simulink model "ControlDigital_Observadores"  (R2016a)
settings: Solver=VariableStepAuto  StartTime=0.0  StopTime=50  RelTol=1e-3
values from neighbouring files (symbols this model uses):
  Ac_2 = [ALn-BLn*Kest-L*CLn+L*DLn*Kest, BLn*Ki - L*DLn*Ki ... (first row only)    [Control_MIMO_Observadores.m]    (also in Diseno_lqg_funcion_transferencia.m = Reg_2dof.a; Ejercicio_funcion_lqg.m = Reg_2dof.a)
  ALn = double(subs(AL,{a,b,c,d},{a1,b1,c1,d1}))    [Control_MIMO_Observadores.m]    (also in Control_MIMO_Observadores_Equilibrio.m)
  Bc_2 = [zeros(n,r),L ... (first row only)    [Control_MIMO_Observadores.m]    (also in Diseno_lqg_funcion_transferencia.m = Reg_2dof.b; Ejercicio_funcion_lqg.m = Reg_2dof.b)
  BLn = double(subs(BL,{a,b,c,d},{a1,b1,c1,d1}))    [Control_MIMO_Observadores.m]    (also in Control_MIMO_Observadores_Equilibrio.m)
  Cc_2 = [-Kest, Ki]    [Control_MIMO_Observadores.m]    (also in Diseno_lqg_funcion_transferencia.m = Reg_2dof.c; Ejercicio_funcion_lqg.m = Reg_2dof.c)
  CLn = [1 0 0 ... (first row only)    [Control_MIMO_Observadores.m]    (also in Control_MIMO_Observadores_Equilibrio.m)
  Dc_2 = zeros(p,2*r)    [Control_MIMO_Observadores.m]    (also in Diseno_lqg_funcion_transferencia.m = Reg_2dof.d; Ejercicio_funcion_lqg.m = Reg_2dof.d)
  DLn = [0 0 0 ... (first row only)    [Control_MIMO_Observadores.m]    (also in Control_MIMO_Observadores_Equilibrio.m)
  Kaw = [0 0 0 ... (first row only)    [Control_MIMO_Observadores.m]
  Kest = Kt(:,1:n)    [Control_MIMO_Observadores.m]
  Ki = -Kt(:,n+1:end)    [Control_MIMO_Observadores.m]
  L = (Grand*inv(X))'    [Control_MIMO_Observadores.m]    (also in Control_MIMO_Observadores_Equilibrio.m)
  sys_d2 = c2d(sys_c2,Tm)    [Control_MIMO_Observadores.m]
  Tm = 0.01    [Control_MIMO_Observadores.m]    (also in Control_MIMO_Observadores_Equilibrio.m)
  u10 = double((a1*x20 + b1*x10^2)/u20)    [Control_MIMO_Observadores.m]    (also in Control_MIMO_Observadores_Equilibrio.m)
  u20 = double(sqrt(c1*x30*x20))    [Control_MIMO_Observadores.m]    (also in Control_MIMO_Observadores_Equilibrio.m)
  u30 = double((d1*x30 - u10)/x10)    [Control_MIMO_Observadores.m]    (also in Control_MIMO_Observadores_Equilibrio.m)
  x10 = 2    [Control_MIMO_Observadores.m]    (also in Control_MIMO_Observadores_Equilibrio.m)
  x20 = 4    [Control_MIMO_Observadores.m]    (also in Control_MIMO_Observadores_Equilibrio.m)
  x30 = 4    [Control_MIMO_Observadores.m]    (also in Control_MIMO_Observadores_Equilibrio.m)
  xini = [0.5; -0.3; -0.7]    [Control_MIMO_Observadores_Equilibrio.m]
libraries: simulink x14, cstblocks x5
settings Model: Creator=Lenovo  LastModifiedBy=Lenovo

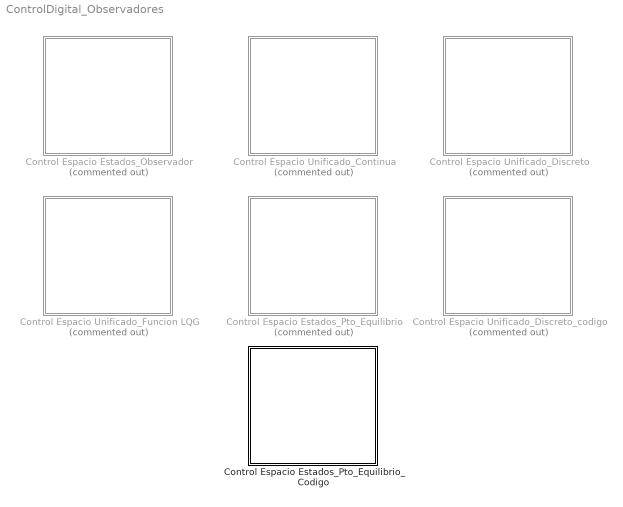
== system ControlDigital_Observadores ==
  Control Espacio Estados_Observador : Subsystem  Commented=on
  Control Espacio Estados_Pto_Equilibrio : Subsystem  Commented=on
  Control Espacio Estados_Pto_Equilibrio_Codigo : Subsystem
  Control Espacio Unificado_Continua : Subsystem  Commented=on
  Control Espacio Unificado_Discreto : Subsystem  Commented=on
  Control Espacio Unificado_Discreto_codigo : Subsystem  Commented=on
  Control Espacio Unificado_Funcion LQG : Subsystem  Commented=on

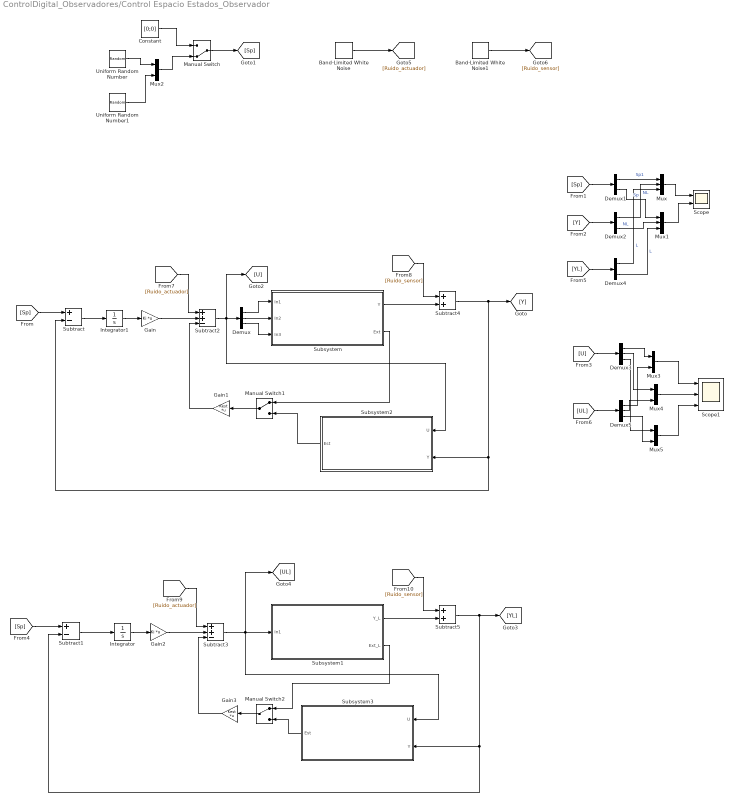
== system ControlDigital_Observadores/Control Espacio Estados_Observador ==
  Band-Limited White Noise : simulink/Sources/Band-Limited White Noise  Cov=[1e-6, 1e-7, 1e-6 ]  Ts=0.01  seed=[23341]
  Band-Limited White Noise1 : simulink/Sources/Band-Limited White Noise  Cov=[1e-6, 1e-6]  Ts=0.01  seed=[23341]
  Constant : Constant  Value=[0;0]
  Demux : Demux  Outputs=3
  Demux1 : Demux  Outputs=2
  Demux2 : Demux  Outputs=2
  Demux3 : Demux  Outputs=3
  Demux4 : Demux  Outputs=2
  Demux5 : Demux  Outputs=3
  Gain : Gain  Gain=Ki  Multiplication=Matrix(K*u)
  Gain1 : Gain  Gain=Kest  Multiplication=Matrix(K*u)
  Gain2 : Gain  Gain=Ki  Multiplication=Matrix(K*u)
  Gain3 : Gain  Gain=Kest  Multiplication=Matrix(K*u)
  Integrator : Integrator
  Integrator1 : Integrator
  Manual Switch : ManualSwitch  CurrentSetting=0
  Manual Switch1 : ManualSwitch
  Manual Switch2 : ManualSwitch
  Mux : Mux  Inputs=3
  Mux1 : Mux  Inputs=3
  Mux{2..5} (4 alike) : Mux  Inputs=2
  Scope : Scope  NumInputPorts=2
  Scope1 : Scope  NumInputPorts=3
  Subsystem : Subsystem
  Subsystem1 : Subsystem
  Subsystem2 : Subsystem
  Subsystem3 : Subsystem
  Subtract : Sum  Inputs=+-
  Subtract1 : Sum  Inputs=+-
  Subtract2 : Sum  Inputs=++-
  Subtract3 : Sum  Inputs=++-
  Subtract4 : Sum
  Subtract5 : Sum
  Uniform Random Number : UniformRandomNumber  Minimum=-0.3  Maximum=0.3  SampleTime=6
  Uniform Random Number1 : UniformRandomNumber  Minimum=-0.5  Maximum=0.5  SampleTime=13
  wires:
  Demux2/1 -> Mux/2  "NL"
  Demux2/2 -> Mux1/2  "NL"
  [Sp] -> Demux1/1
  [Sp] -> Subtract/1
  Demux/3 -> Subsystem/3(In3)
  Demux/2 -> Subsystem/2(In2)
  Constant/1 -> Manual Switch/1
  Manual Switch/1 -> [Sp]
  Demux1/1 -> Mux/1  "Sp1"
  Demux1/2 -> Mux1/1  "Sp"
  Demux/1 -> Subsystem/1(In1)
  [Y] -> Demux2/1
  Mux1/1 -> Scope/2
  Mux/1 -> Scope/1
  Mux5/1 -> Scope1/3
  Uniform Random Number/1 -> Mux2/1
  [Sp] -> Subtract1/1
  Demux5/1 -> Mux3/2
  [U] -> Demux3/1
  Demux5/3 -> Mux5/2
  [YL] -> Demux4/1
  Demux3/2 -> Mux4/1
  Demux3/1 -> Mux3/1
  Demux3/3 -> Mux5/1
  Demux5/2 -> Mux4/2
  Mux3/1 -> Scope1/1
  Mux4/1 -> Scope1/2
  Demux4/2 -> Mux1/3  "L"
  Uniform Random Number1/1 -> Mux2/2
  Demux4/1 -> Mux/3  "L"
  [UL] -> Demux5/1
  Mux2/1 -> Manual Switch/2
  Subtract2/1 -> Subsystem2/1(U), [U], Demux/1
  Manual Switch1/1 -> Gain1/1
  Subsystem/2(Ext) -> Manual Switch1/1
  Subsystem2/1(Est) -> Manual Switch1/2
  Subsystem3/1(Est) -> Manual Switch2/2
  Subsystem1/2(Ext_L) -> Manual Switch2/1
  Subtract1/1 -> Integrator/1
  Integrator1/1 -> Gain/1
  Subtract/1 -> Integrator1/1
  Band-Limited White Noise/1 -> [Ruido_actuador]
  Band-Limited White Noise1/1 -> [Ruido_sensor]
  Gain1/1 -> Subtract2/3
  Gain/1 -> Subtract2/2
  [Ruido_actuador] -> Subtract2/1
  Subtract4/1 -> [Y], Subsystem2/2(Y), Subtract/2
  Subsystem/1(Y) -> Subtract4/2
  [Ruido_sensor] -> Subtract4/1
  Subtract3/1 -> Subsystem3/1(U), [UL], Subsystem1/1(In1)
  Integrator/1 -> Gain2/1
  Gain3/1 -> Subtract3/3
  Gain2/1 -> Subtract3/2
  [Ruido_actuador] -> Subtract3/1
  Manual Switch2/1 -> Gain3/1
  Subsystem1/1(Y_L) -> Subtract5/2
  [Ruido_sensor] -> Subtract5/1
  Subtract5/1 -> Subsystem3/2(Y), Subtract1/2, [YL]

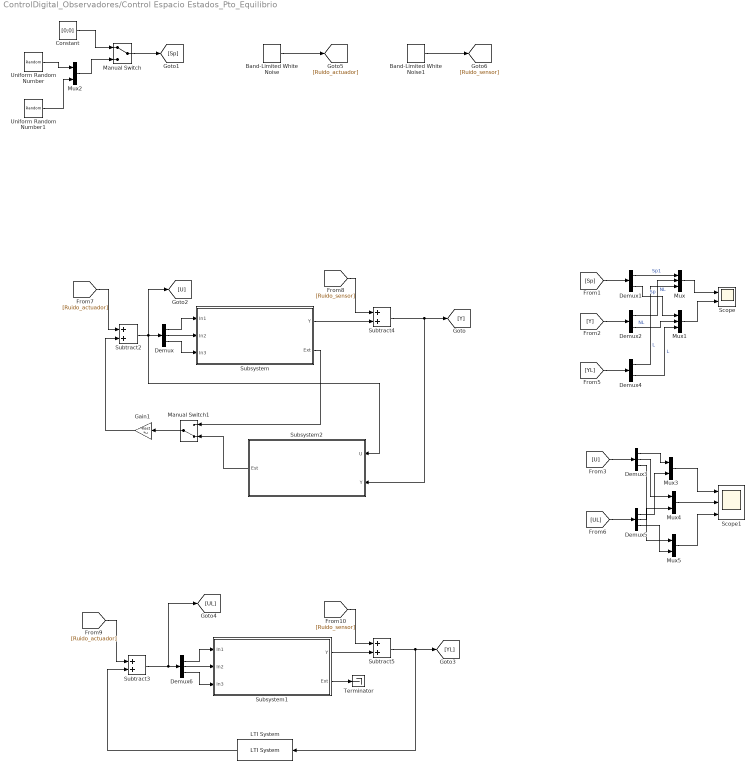
== system ControlDigital_Observadores/Control Espacio Estados_Pto_Equilibrio ==
  Band-Limited White Noise : simulink/Sources/Band-Limited White Noise  Cov=[1e-7, 1e-8, 1e-7 ]  Ts=1e-3  seed=[23341]
  Band-Limited White Noise1 : simulink/Sources/Band-Limited White Noise  Cov=[1e-7, 1e-7]  Ts=1e-3  seed=[23341]
  Constant : Constant  Value=[0;0]
  Demux{,3,5..6} (4 alike) : Demux  Outputs=3
  Demux1 : Demux  Outputs=2
  Demux2 : Demux  Outputs=2
  Demux4 : Demux  Outputs=2
  Gain1 : Gain  Gain=-Kest  Multiplication=Matrix(K*u)
  LTI System : cstblocks/LTI System  sys=sys_c_dig  IC=[]
  Manual Switch : ManualSwitch
  Manual Switch1 : ManualSwitch  CurrentSetting=0
  Mux : Mux  Inputs=3
  Mux1 : Mux  Inputs=3
  Mux{2..5} (4 alike) : Mux  Inputs=2
  Scope : Scope  NumInputPorts=2
  Scope1 : Scope  NumInputPorts=3
  Subsystem : Subsystem
  Subsystem1 : Subsystem
  Subsystem2 : Subsystem
  Subtract{2..5} (4 alike) : Sum
  Terminator : Terminator
  Uniform Random Number : UniformRandomNumber  Minimum=-0.3  Maximum=0.3  SampleTime=6
  Uniform Random Number1 : UniformRandomNumber  Minimum=-0.5  Maximum=0.5  SampleTime=13
  wires:
  Demux2/1 -> Mux/2  "NL"
  Demux2/2 -> Mux1/2  "NL"
  [Sp] -> Demux1/1
  Demux/3 -> Subsystem/3(In3)
  Demux/2 -> Subsystem/2(In2)
  Constant/1 -> Manual Switch/1
  Manual Switch/1 -> [Sp]
  Demux1/1 -> Mux/1  "Sp1"
  Demux1/2 -> Mux1/1  "Sp"
  Demux/1 -> Subsystem/1(In1)
  [Y] -> Demux2/1
  Mux1/1 -> Scope/2
  Mux/1 -> Scope/1
  Mux5/1 -> Scope1/3
  Uniform Random Number/1 -> Mux2/1
  Demux5/1 -> Mux3/2
  [U] -> Demux3/1
  Demux5/3 -> Mux5/2
  [YL] -> Demux4/1
  Demux3/2 -> Mux4/1
  Demux3/1 -> Mux3/1
  Demux3/3 -> Mux5/1
  Demux5/2 -> Mux4/2
  Mux3/1 -> Scope1/1
  Mux4/1 -> Scope1/2
  Demux4/2 -> Mux1/3  "L"
  Uniform Random Number1/1 -> Mux2/2
  Demux4/1 -> Mux/3  "L"
  [UL] -> Demux5/1
  Mux2/1 -> Manual Switch/2
  Subtract2/1 -> Subsystem2/1(U), [U], Demux/1
  Manual Switch1/1 -> Gain1/1
  Subsystem/2(Ext) -> Manual Switch1/1
  Subsystem2/1(Est) -> Manual Switch1/2
  Band-Limited White Noise/1 -> [Ruido_actuador]
  Band-Limited White Noise1/1 -> [Ruido_sensor]
  [Ruido_actuador] -> Subtract2/1
  Subtract4/1 -> [Y], Subsystem2/2(Y)
  Subsystem/1(Y) -> Subtract4/2
  [Ruido_sensor] -> Subtract4/1
  Subtract3/1 -> Demux6/1, [UL]
  [Ruido_actuador] -> Subtract3/1
  [Ruido_sensor] -> Subtract5/1
  Subtract5/1 -> LTI System/1, [YL]
  Gain1/1 -> Subtract2/2
  Subsystem1/2(Ext) -> Terminator/1
  LTI System/1 -> Subtract3/2
  Demux6/3 -> Subsystem1/3(In3)
  Demux6/2 -> Subsystem1/2(In2)
  Demux6/1 -> Subsystem1/1(In1)
  Subsystem1/1(Y) -> Subtract5/2

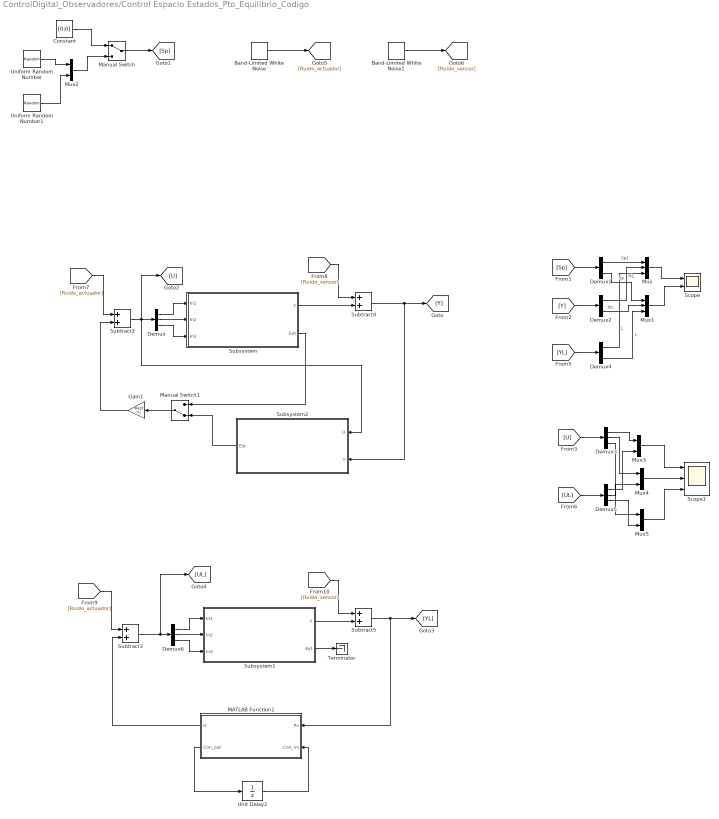
== system ControlDigital_Observadores/Control Espacio Estados_Pto_Equilibrio_Codigo ==
  Band-Limited White Noise : simulink/Sources/Band-Limited White Noise  Cov=[1e-7, 1e-8, 1e-7 ]  Ts=1e-3  seed=[23341]
  Band-Limited White Noise1 : simulink/Sources/Band-Limited White Noise  Cov=[1e-7, 1e-7]  Ts=1e-3  seed=[23341]
  Constant : Constant  Value=[0;0]
  Demux{,3,5..6} (4 alike) : Demux  Outputs=3
  Demux1 : Demux  Outputs=2
  Demux2 : Demux  Outputs=2
  Demux4 : Demux  Outputs=2
  Gain1 : Gain  Gain=-Kest  Multiplication=Matrix(K*u)
  MATLAB Function1 : MATLAB Function  TreatAsAtomicUnit=on
  Manual Switch : ManualSwitch
  Manual Switch1 : ManualSwitch  CurrentSetting=0
  Mux : Mux  Inputs=3
  Mux1 : Mux  Inputs=3
  Mux{2..5} (4 alike) : Mux  Inputs=2
  Scope : Scope  NumInputPorts=2
  Scope1 : Scope  NumInputPorts=3
  Subsystem : Subsystem
  Subsystem1 : Subsystem
  Subsystem2 : Subsystem
  Subtract{2..5} (4 alike) : Sum
  Terminator : Terminator
  Uniform Random Number : UniformRandomNumber  Minimum=-0.3  Maximum=0.3  SampleTime=6
  Uniform Random Number1 : UniformRandomNumber  Minimum=-0.5  Maximum=0.5  SampleTime=13
  Unit Delay2 : UnitDelay  InitialCondition=zeros(3,1)  SampleTime=Tm
  wires:
  Demux2/1 -> Mux/2  "NL"
  Demux2/2 -> Mux1/2  "NL"
  [Sp] -> Demux1/1
  Demux/3 -> Subsystem/3(In3)
  Demux/2 -> Subsystem/2(In2)
  Constant/1 -> Manual Switch/1
  Manual Switch/1 -> [Sp]
  Demux1/1 -> Mux/1  "Sp1"
  Demux1/2 -> Mux1/1  "Sp"
  Demux/1 -> Subsystem/1(In1)
  [Y] -> Demux2/1
  Mux1/1 -> Scope/2
  Mux/1 -> Scope/1
  Mux5/1 -> Scope1/3
  Uniform Random Number/1 -> Mux2/1
  Demux5/1 -> Mux3/2
  [U] -> Demux3/1
  Demux5/3 -> Mux5/2
  [YL] -> Demux4/1
  Demux3/2 -> Mux4/1
  Demux3/1 -> Mux3/1
  Demux3/3 -> Mux5/1
  Demux5/2 -> Mux4/2
  Mux3/1 -> Scope1/1
  Mux4/1 -> Scope1/2
  Demux4/2 -> Mux1/3  "L"
  Uniform Random Number1/1 -> Mux2/2
  Demux4/1 -> Mux/3  "L"
  [UL] -> Demux5/1
  Mux2/1 -> Manual Switch/2
  Subtract2/1 -> Subsystem2/1(U), [U], Demux/1
  Manual Switch1/1 -> Gain1/1
  Subsystem/2(Ext) -> Manual Switch1/1
  Subsystem2/1(Est) -> Manual Switch1/2
  Band-Limited White Noise/1 -> [Ruido_actuador]
  Band-Limited White Noise1/1 -> [Ruido_sensor]
  [Ruido_actuador] -> Subtract2/1
  Subtract4/1 -> [Y], Subsystem2/2(Y)
  Subsystem/1(Y) -> Subtract4/2
  [Ruido_sensor] -> Subtract4/1
  Subtract3/1 -> Demux6/1, [UL]
  [Ruido_actuador] -> Subtract3/1
  [Ruido_sensor] -> Subtract5/1
  Subtract5/1 -> MATLAB Function1/1(Pv), [YL]
  Gain1/1 -> Subtract2/2
  Subsystem1/2(Ext) -> Terminator/1
  Demux6/3 -> Subsystem1/3(In3)
  Demux6/2 -> Subsystem1/2(In2)
  Demux6/1 -> Subsystem1/1(In1)
  Subsystem1/1(Y) -> Subtract5/2
  MATLAB Function1/1(U) -> Subtract3/2
  MATLAB Function1/2(Con_out) -> Unit Delay2/1
  Unit Delay2/1 -> MATLAB Function1/2(Con_ini)

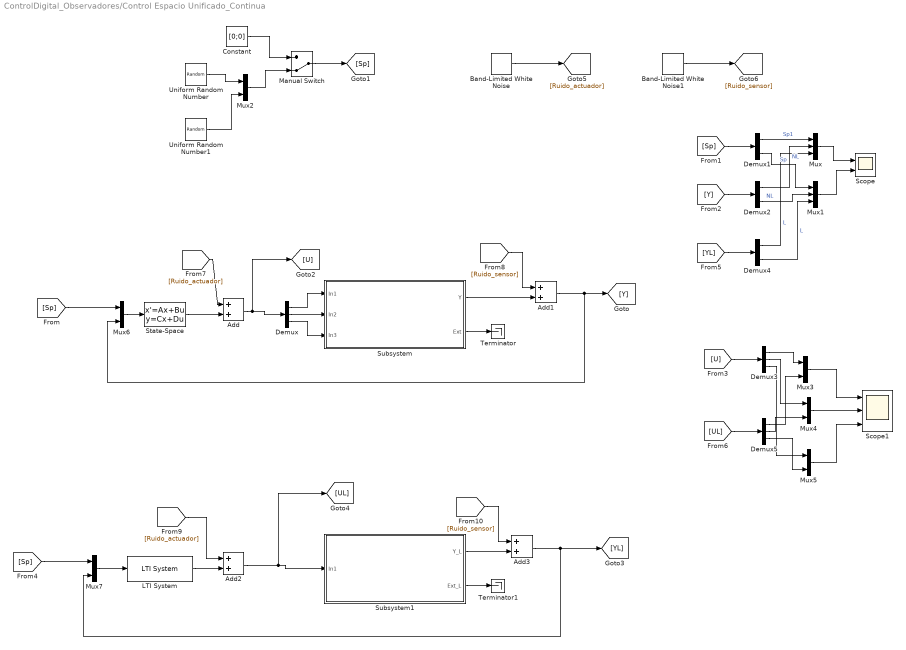
== system ControlDigital_Observadores/Control Espacio Unificado_Continua ==
  Add{,1..3} (4 alike) : Sum
  Band-Limited White Noise : simulink/Sources/Band-Limited White Noise  Cov=[1e-6, 1e-7, 1e-6 ]  Ts=0.01  seed=[23341]
  Band-Limited White Noise1 : simulink/Sources/Band-Limited White Noise  Cov=[1e-6, 1e-6]  Ts=0.01  seed=[23341]
  Constant : Constant  Value=[0;0]
  Demux : Demux  Outputs=3
  Demux1 : Demux  Outputs=2
  Demux2 : Demux  Outputs=2
  Demux3 : Demux  Outputs=3
  Demux4 : Demux  Outputs=2
  Demux5 : Demux  Outputs=3
  LTI System : cstblocks/LTI System  sys=sys_c2  IC=[]
  Manual Switch : ManualSwitch  CurrentSetting=0
  Mux : Mux  Inputs=3
  Mux1 : Mux  Inputs=3
  Mux{2..7} (6 alike) : Mux  Inputs=2
  Scope : Scope  NumInputPorts=2
  Scope1 : Scope  NumInputPorts=3
  State-Space : StateSpace  A=Ac_2  B=Bc_2  C=Cc_2  D=Dc_2  X0=0
  Subsystem : Subsystem
  Subsystem1 : Subsystem
  Terminator : Terminator
  Terminator1 : Terminator
  Uniform Random Number : UniformRandomNumber  Minimum=-0.3  Maximum=0.3  SampleTime=6
  Uniform Random Number1 : UniformRandomNumber  Minimum=-0.5  Maximum=0.5  SampleTime=13
  wires:
  Demux2/1 -> Mux/2  "NL"
  Demux2/2 -> Mux1/2  "NL"
  [Sp] -> Demux1/1
  Demux/3 -> Subsystem/3(In3)
  Demux/2 -> Subsystem/2(In2)
  Constant/1 -> Manual Switch/1
  Manual Switch/1 -> [Sp]
  Demux1/1 -> Mux/1  "Sp1"
  Demux1/2 -> Mux1/1  "Sp"
  Demux/1 -> Subsystem/1(In1)
  [Y] -> Demux2/1
  Mux1/1 -> Scope/2
  Mux/1 -> Scope/1
  Mux5/1 -> Scope1/3
  Uniform Random Number/1 -> Mux2/1
  Demux5/1 -> Mux3/2
  [U] -> Demux3/1
  Demux5/3 -> Mux5/2
  [YL] -> Demux4/1
  Demux3/2 -> Mux4/1
  Demux3/1 -> Mux3/1
  Demux3/3 -> Mux5/1
  Demux5/2 -> Mux4/2
  Mux3/1 -> Scope1/1
  Mux4/1 -> Scope1/2
  Demux4/2 -> Mux1/3  "L"
  Uniform Random Number1/1 -> Mux2/2
  Demux4/1 -> Mux/3  "L"
  [UL] -> Demux5/1
  Mux2/1 -> Manual Switch/2
  Subsystem/2(Ext) -> Terminator/1
  Mux6/1 -> State-Space/1
  [Sp] -> Mux6/1
  [Sp] -> Mux7/1
  Subsystem1/2(Ext_L) -> Terminator1/1
  Band-Limited White Noise/1 -> [Ruido_actuador]
  Band-Limited White Noise1/1 -> [Ruido_sensor]
  State-Space/1 -> Add/2
  Add/1 -> [U], Demux/1
  [Ruido_actuador] -> Add/1
  Subsystem/1(Y) -> Add1/2
  Add1/1 -> Mux6/2, [Y]
  [Ruido_sensor] -> Add1/1
  LTI System/1 -> Add2/2
  [Ruido_actuador] -> Add2/1
  Add2/1 -> [UL], Subsystem1/1(In1)
  Add3/1 -> Mux7/2, [YL]
  [Ruido_sensor] -> Add3/1
  Subsystem1/1(Y_L) -> Add3/2
  Mux7/1 -> LTI System/1

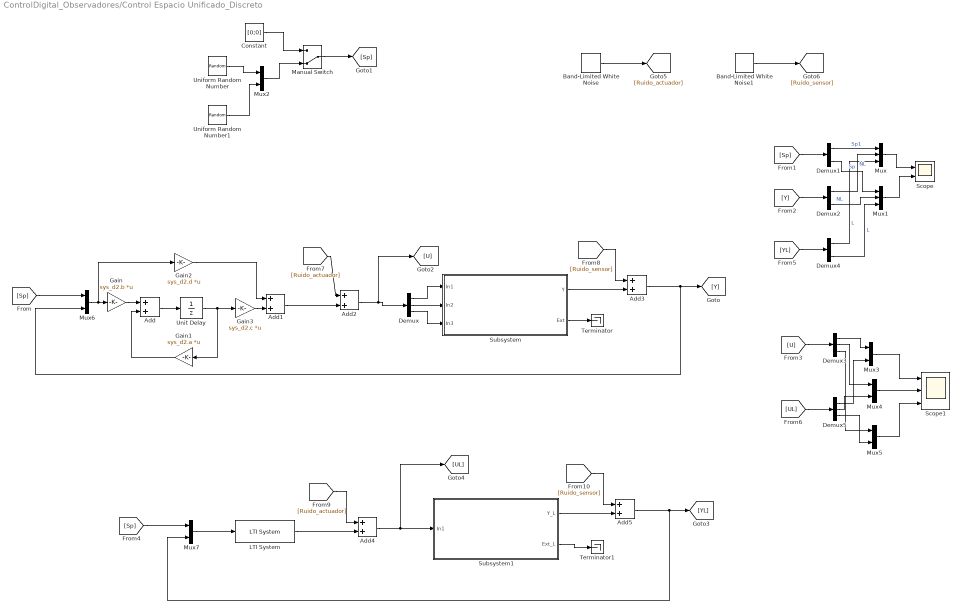
== system ControlDigital_Observadores/Control Espacio Unificado_Discreto ==
  Add{,1..5} (6 alike) : Sum
  Band-Limited White Noise : simulink/Sources/Band-Limited White Noise  Cov=[1e-6, 1e-7, 1e-6 ]  Ts=0.01  seed=[23341]
  Band-Limited White Noise1 : simulink/Sources/Band-Limited White Noise  Cov=[1e-6, 1e-6]  Ts=0.01  seed=[23341]
  Constant : Constant  Value=[0;0]
  Demux : Demux  Outputs=3
  Demux1 : Demux  Outputs=2
  Demux2 : Demux  Outputs=2
  Demux3 : Demux  Outputs=3
  Demux4 : Demux  Outputs=2
  Demux5 : Demux  Outputs=3
  Gain : Gain  Gain=sys_d2.b  Multiplication=Matrix(K*u)
  Gain1 : Gain  Gain=sys_d2.a  Multiplication=Matrix(K*u)
  Gain2 : Gain  Gain=sys_d2.d  Multiplication=Matrix(K*u)
  Gain3 : Gain  Gain=sys_d2.c  Multiplication=Matrix(K*u)
  LTI System : cstblocks/LTI System  sys=sys_d2  IC=[]
  Manual Switch : ManualSwitch  CurrentSetting=0
  Mux : Mux  Inputs=3
  Mux1 : Mux  Inputs=3
  Mux{2..7} (6 alike) : Mux  Inputs=2
  Scope : Scope  NumInputPorts=2
  Scope1 : Scope  NumInputPorts=3
  Subsystem : Subsystem
  Subsystem1 : Subsystem
  Terminator : Terminator
  Terminator1 : Terminator
  Uniform Random Number : UniformRandomNumber  Minimum=-0.3  Maximum=0.3  SampleTime=6
  Uniform Random Number1 : UniformRandomNumber  Minimum=-0.5  Maximum=0.5  SampleTime=13
  Unit Delay : UnitDelay  SampleTime=Tm
  wires:
  Demux2/1 -> Mux/2  "NL"
  Demux2/2 -> Mux1/2  "NL"
  [Sp] -> Demux1/1
  Demux/3 -> Subsystem/3(In3)
  Demux/2 -> Subsystem/2(In2)
  Constant/1 -> Manual Switch/1
  Manual Switch/1 -> [Sp]
  Demux1/1 -> Mux/1  "Sp1"
  Demux1/2 -> Mux1/1  "Sp"
  Demux/1 -> Subsystem/1(In1)
  [Y] -> Demux2/1
  Mux1/1 -> Scope/2
  Mux/1 -> Scope/1
  Mux5/1 -> Scope1/3
  Uniform Random Number/1 -> Mux2/1
  Demux5/1 -> Mux3/2
  [U] -> Demux3/1
  Demux5/3 -> Mux5/2
  [YL] -> Demux4/1
  Demux3/2 -> Mux4/1
  Demux3/1 -> Mux3/1
  Demux3/3 -> Mux5/1
  Demux5/2 -> Mux4/2
  Mux3/1 -> Scope1/1
  Mux4/1 -> Scope1/2
  Demux4/2 -> Mux1/3  "L"
  Uniform Random Number1/1 -> Mux2/2
  Demux4/1 -> Mux/3  "L"
  [UL] -> Demux5/1
  Mux2/1 -> Manual Switch/2
  Subsystem/2(Ext) -> Terminator/1
  [Sp] -> Mux6/1
  Mux7/1 -> LTI System/1
  [Sp] -> Mux7/1
  Subsystem1/2(Ext_L) -> Terminator1/1
  Mux6/1 -> Gain2/1, Gain/1
  Gain/1 -> Add/1
  Add/1 -> Unit Delay/1
  Unit Delay/1 -> Gain3/1, Gain1/1
  Gain1/1 -> Add/2
  Gain2/1 -> Add1/1
  Gain3/1 -> Add1/2
  Add1/1 -> Add2/2
  [Ruido_actuador] -> Add2/1
  Add2/1 -> [U], Demux/1
  Subsystem/1(Y) -> Add3/2
  [Ruido_sensor] -> Add3/1
  Add3/1 -> Mux6/2, [Y]
  LTI System/1 -> Add4/2
  [Ruido_actuador] -> Add4/1
  Add4/1 -> [UL], Subsystem1/1(In1)
  Subsystem1/1(Y_L) -> Add5/2
  [Ruido_sensor] -> Add5/1
  Add5/1 -> Mux7/2, [YL]
  Band-Limited White Noise/1 -> [Ruido_actuador]
  Band-Limited White Noise1/1 -> [Ruido_sensor]

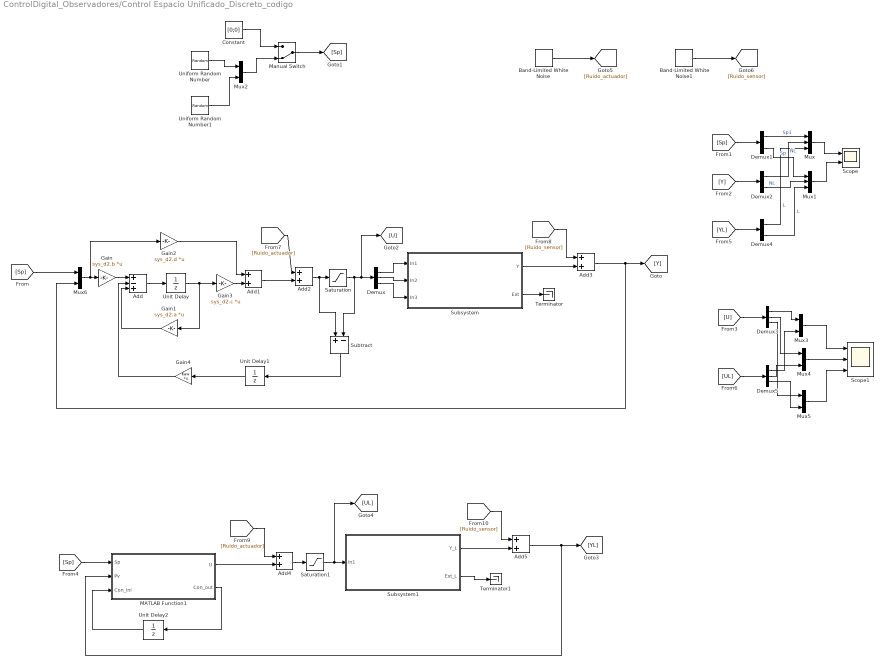
== system ControlDigital_Observadores/Control Espacio Unificado_Discreto_codigo ==
  Add : Sum  Inputs=+-+
  Add{1..5} (5 alike) : Sum
  Band-Limited White Noise : simulink/Sources/Band-Limited White Noise  Cov=[1e-6, 1e-7, 1e-6 ]  Ts=0.01  seed=[23341]
  Band-Limited White Noise1 : simulink/Sources/Band-Limited White Noise  Cov=[1e-7, 1e-7]  Ts=0.01  seed=[23341]
  Constant : Constant  Value=[0;0]
  Demux : Demux  Outputs=3
  Demux1 : Demux  Outputs=2
  Demux2 : Demux  Outputs=2
  Demux3 : Demux  Outputs=3
  Demux4 : Demux  Outputs=2
  Demux5 : Demux  Outputs=3
  Gain : Gain  Gain=sys_d2.b  Multiplication=Matrix(K*u)
  Gain1 : Gain  Gain=sys_d2.a  Multiplication=Matrix(K*u)
  Gain2 : Gain  Gain=sys_d2.d  Multiplication=Matrix(K*u)
  Gain3 : Gain  Gain=sys_d2.c  Multiplication=Matrix(K*u)
  Gain4 : Gain  Gain=Kaw  Multiplication=Matrix(K*u)
  MATLAB Function1 : MATLAB Function  TreatAsAtomicUnit=on
  Manual Switch : ManualSwitch  CurrentSetting=0
  Mux : Mux  Inputs=3
  Mux1 : Mux  Inputs=3
  Mux{2..6} (5 alike) : Mux  Inputs=2
  Saturation : Saturate  UpperLimit=[2; 2;2]  LowerLimit=[-2; -2;-2]
  Saturation1 : Saturate  UpperLimit=[2; 2;2]  LowerLimit=[-2; -2;-2]
  Scope : Scope  NumInputPorts=2
  Scope1 : Scope  NumInputPorts=3
  Subsystem : Subsystem
  Subsystem1 : Subsystem
  Subtract : Sum  Inputs=+-
  Terminator : Terminator
  Terminator1 : Terminator
  Uniform Random Number : UniformRandomNumber  Minimum=-0.3  Maximum=0.3  SampleTime=6
  Uniform Random Number1 : UniformRandomNumber  Minimum=-0.5  Maximum=0.5  SampleTime=13
  Unit Delay : UnitDelay  SampleTime=Tm
  Unit Delay1 : UnitDelay  SampleTime=Tm
  Unit Delay2 : UnitDelay  InitialCondition=zeros(5,1)  SampleTime=Tm
  wires:
  Demux2/1 -> Mux/2  "NL"
  Demux2/2 -> Mux1/2  "NL"
  [Sp] -> Demux1/1
  Demux/3 -> Subsystem/3(In3)
  Demux/2 -> Subsystem/2(In2)
  Constant/1 -> Manual Switch/1
  Manual Switch/1 -> [Sp]
  Demux1/1 -> Mux/1  "Sp1"
  Demux1/2 -> Mux1/1  "Sp"
  Demux/1 -> Subsystem/1(In1)
  [Y] -> Demux2/1
  Mux1/1 -> Scope/2
  Mux/1 -> Scope/1
  Mux5/1 -> Scope1/3
  Uniform Random Number/1 -> Mux2/1
  Demux5/1 -> Mux3/2
  [U] -> Demux3/1
  Demux5/3 -> Mux5/2
  [YL] -> Demux4/1
  Demux3/2 -> Mux4/1
  Demux3/1 -> Mux3/1
  Demux3/3 -> Mux5/1
  Demux5/2 -> Mux4/2
  Mux3/1 -> Scope1/1
  Mux4/1 -> Scope1/2
  Demux4/2 -> Mux1/3  "L"
  Uniform Random Number1/1 -> Mux2/2
  Demux4/1 -> Mux/3  "L"
  [UL] -> Demux5/1
  Mux2/1 -> Manual Switch/2
  Subsystem/2(Ext) -> Terminator/1
  [Sp] -> Mux6/1
  Subsystem1/2(Ext_L) -> Terminator1/1
  Mux6/1 -> Gain2/1, Gain/1
  Gain/1 -> Add/1
  Add/1 -> Unit Delay/1
  Unit Delay/1 -> Gain3/1, Gain1/1
  Gain2/1 -> Add1/1
  Gain3/1 -> Add1/2
  Add1/1 -> Add2/2
  [Ruido_actuador] -> Add2/1
  Subsystem/1(Y) -> Add3/2
  [Ruido_sensor] -> Add3/1
  Add3/1 -> Mux6/2, [Y]
  MATLAB Function1/1(U) -> Add4/2
  [Ruido_actuador] -> Add4/1
  Add4/1 -> Saturation1/1
  Subsystem1/1(Y_L) -> Add5/2
  [Ruido_sensor] -> Add5/1
  Add5/1 -> MATLAB Function1/2(Pv), [YL]
  Band-Limited White Noise/1 -> [Ruido_actuador]
  Band-Limited White Noise1/1 -> [Ruido_sensor]
  Add2/1 -> Subtract/1, Saturation/1
  Saturation/1 -> Subtract/2, [U], Demux/1
  Subtract/1 -> Unit Delay1/1
  Unit Delay1/1 -> Gain4/1
  Gain1/1 -> Add/3
  Gain4/1 -> Add/2
  [Sp] -> MATLAB Function1/1(Sp)
  Unit Delay2/1 -> MATLAB Function1/3(Con_ini)
  MATLAB Function1/2(Con_out) -> Unit Delay2/1
  Saturation1/1 -> [UL], Subsystem1/1(In1)

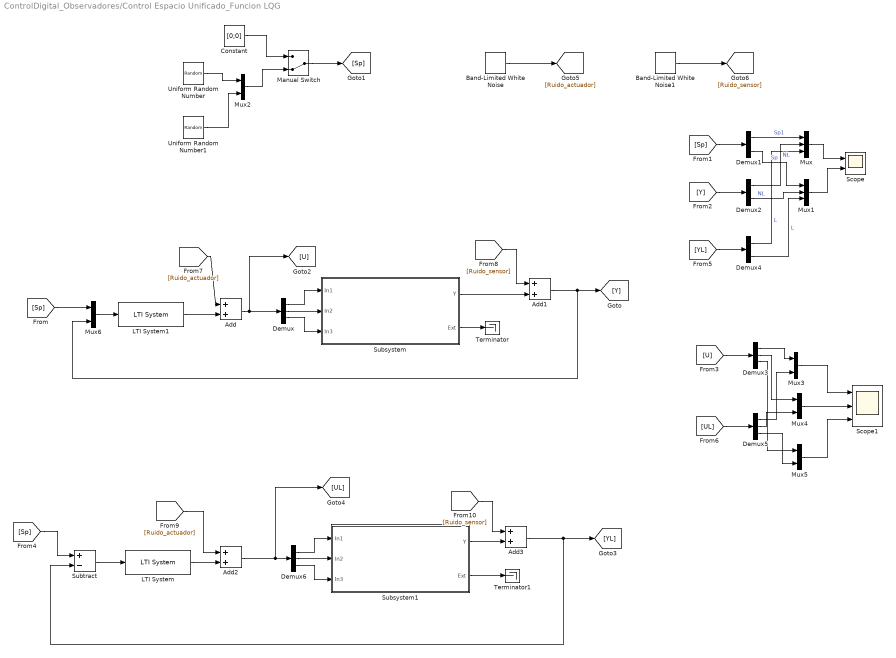
== system ControlDigital_Observadores/Control Espacio Unificado_Funcion LQG ==
  Add{,1..3} (4 alike) : Sum
  Band-Limited White Noise : simulink/Sources/Band-Limited White Noise  Cov=[1e-6, 1e-7, 1e-6 ]  Ts=0.01  seed=[23341]
  Band-Limited White Noise1 : simulink/Sources/Band-Limited White Noise  Cov=[1e-6, 1e-6]  Ts=0.01  seed=[23341]
  Constant : Constant  Value=[0;0]
  Demux{,3,5..6} (4 alike) : Demux  Outputs=3
  Demux1 : Demux  Outputs=2
  Demux2 : Demux  Outputs=2
  Demux4 : Demux  Outputs=2
  LTI System : cstblocks/LTI System  sys=Reg_1dof  IC=[]
  LTI System1 : cstblocks/LTI System  sys=Reg_2dof  IC=[]
  Manual Switch : ManualSwitch  CurrentSetting=0
  Mux : Mux  Inputs=3
  Mux1 : Mux  Inputs=3
  Mux{2..6} (5 alike) : Mux  Inputs=2
  Scope : Scope  NumInputPorts=2
  Scope1 : Scope  NumInputPorts=3
  Subsystem : Subsystem
  Subsystem1 : Subsystem
  Subtract : Sum  Inputs=+-
  Terminator : Terminator
  Terminator1 : Terminator
  Uniform Random Number : UniformRandomNumber  Minimum=-0.4  Maximum=0.4  SampleTime=6
  Uniform Random Number1 : UniformRandomNumber  Minimum=-0.6  Maximum=0.6  SampleTime=13
  wires:
  Demux2/1 -> Mux/2  "NL"
  Demux2/2 -> Mux1/2  "NL"
  [Sp] -> Demux1/1
  Demux/3 -> Subsystem/3(In3)
  Demux/2 -> Subsystem/2(In2)
  Constant/1 -> Manual Switch/1
  Manual Switch/1 -> [Sp]
  Demux1/1 -> Mux/1  "Sp1"
  Demux1/2 -> Mux1/1  "Sp"
  Demux/1 -> Subsystem/1(In1)
  [Y] -> Demux2/1
  Mux1/1 -> Scope/2
  Mux/1 -> Scope/1
  Mux5/1 -> Scope1/3
  Uniform Random Number/1 -> Mux2/1
  Demux5/1 -> Mux3/2
  [U] -> Demux3/1
  Demux5/3 -> Mux5/2
  [YL] -> Demux4/1
  Demux3/2 -> Mux4/1
  Demux3/1 -> Mux3/1
  Demux3/3 -> Mux5/1
  Demux5/2 -> Mux4/2
  Mux3/1 -> Scope1/1
  Mux4/1 -> Scope1/2
  Demux4/2 -> Mux1/3  "L"
  Uniform Random Number1/1 -> Mux2/2
  Demux4/1 -> Mux/3  "L"
  [UL] -> Demux5/1
  Mux2/1 -> Manual Switch/2
  Subsystem/2(Ext) -> Terminator/1
  Mux6/1 -> LTI System1/1
  [Sp] -> Mux6/1
  Band-Limited White Noise/1 -> [Ruido_actuador]
  Band-Limited White Noise1/1 -> [Ruido_sensor]
  LTI System1/1 -> Add/2
  Add/1 -> [U], Demux/1
  [Ruido_actuador] -> Add/1
  Subsystem/1(Y) -> Add1/2
  Add1/1 -> Mux6/2, [Y]
  [Ruido_sensor] -> Add1/1
  LTI System/1 -> Add2/2
  [Ruido_actuador] -> Add2/1
  Add2/1 -> Demux6/1, [UL]
  Add3/1 -> Subtract/2, [YL]
  [Ruido_sensor] -> Add3/1
  Subtract/1 -> LTI System/1
  [Sp] -> Subtract/1
  Demux6/1 -> Subsystem1/1(In1)
  Subsystem1/1(Y) -> Add3/2
  Subsystem1/2(Ext) -> Terminator1/1
  Demux6/2 -> Subsystem1/2(In2)
  Demux6/3 -> Subsystem1/3(In3)

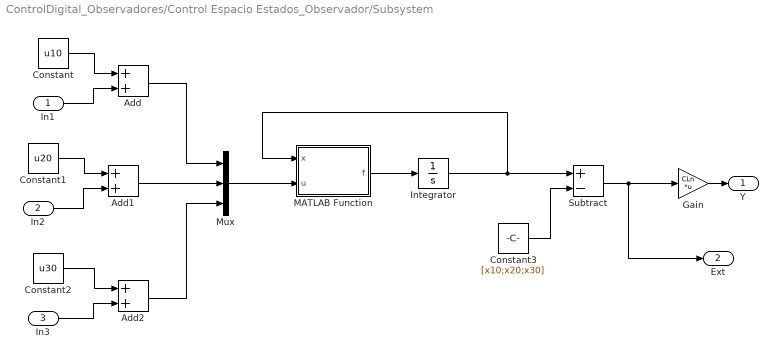
== system ControlDigital_Observadores/Control Espacio Estados_Observador/Subsystem ==
  In1 : Inport
  In2 : Inport  Port=2
  In3 : Inport  Port=3
  Add : Sum
  Add1 : Sum
  Add2 : Sum
  Constant : Constant  Value=u10
  Constant1 : Constant  Value=u20
  Constant2 : Constant  Value=u30
  Constant3 : Constant  Value=[x10;x20;x30]
  Gain : Gain  Gain=CLn  Multiplication=Matrix(K*u)
  Integrator : Integrator  InitialCondition=[x10;x20;x30]
  MATLAB Function : MATLAB Function  TreatAsAtomicUnit=on
  Mux : Mux  Inputs=3
  Subtract : Sum  Inputs=+-
  Y : Outport
  Ext : Outport  Port=2
  wires:
  Subtract/1 -> Ext/1, Gain/1
  Gain/1 -> Y/1
  In1/1 -> Add/2
  Constant/1 -> Add/1
  Add/1 -> Mux/1
  Constant1/1 -> Add1/1
  Add1/1 -> Mux/2
  Mux/1 -> MATLAB Function/2(u)
  Integrator/1 -> MATLAB Function/1(x), Subtract/1
  MATLAB Function/1(f) -> Integrator/1
  In2/1 -> Add1/2
  In3/1 -> Add2/2
  Constant2/1 -> Add2/1
  Constant3/1 -> Subtract/2
  Add2/1 -> Mux/3

== system ControlDigital_Observadores/Control Espacio Estados_Observador/Subsystem1 ==
  In1 : Inport
  Gain1 : Gain  Gain=ALn  Multiplication=Matrix(K*u)
  Gain2 : Gain  Gain=BLn  Multiplication=Matrix(K*u)
  Gain3 : Gain  Gain=DLn  Multiplication=Matrix(K*u)
  Gain4 : Gain  Gain=CLn  Multiplication=Matrix(K*u)
  Integrator : Integrator
  Subtract1 : Sum
  Subtract2 : Sum
  Y_L : Outport
  Ext_L : Outport  Port=2
  wires:
  Subtract2/1 -> Y_L/1
  Subtract1/1 -> Integrator/1
  Integrator/1 -> Ext_L/1, Gain1/1, Gain4/1
  Gain1/1 -> Subtract1/2
  Gain2/1 -> Subtract1/1
  Gain4/1 -> Subtract2/2
  Gain3/1 -> Subtract2/1
  In1/1 -> Gain3/1, Gain2/1

== system ControlDigital_Observadores/Control Espacio Estados_Observador/Subsystem2 ==
  U : Inport
  Y : Inport  Port=2
  Gain1 : Gain  Gain=ALn  Multiplication=Matrix(K*u)
  Gain2 : Gain  Gain=BLn  Multiplication=Matrix(K*u)
  Gain3 : Gain  Gain=DLn  Multiplication=Matrix(K*u)
  Gain4 : Gain  Gain=CLn  Multiplication=Matrix(K*u)
  Gain5 : Gain  Gain=L  Multiplication=Matrix(K*u)
  Integrator : Integrator
  Subtract1 : Sum  Inputs=+++
  Subtract2 : Sum
  Subtract3 : Sum  Inputs=+-
  Est : Outport
  wires:
  Integrator/1 -> Est/1, Gain1/1, Gain4/1
  Gain2/1 -> Subtract1/1
  Gain4/1 -> Subtract2/2
  Gain3/1 -> Subtract2/1
  U/1 -> Gain3/1, Gain2/1
  Y/1 -> Subtract3/1
  Subtract2/1 -> Subtract3/2
  Subtract3/1 -> Gain5/1
  Gain1/1 -> Subtract1/3
  Gain5/1 -> Subtract1/2
  Subtract1/1 -> Integrator/1

== system ControlDigital_Observadores/Control Espacio Estados_Observador/Subsystem3 ==
  U : Inport
  Y : Inport  Port=2
  Gain1 : Gain  Gain=ALn  Multiplication=Matrix(K*u)
  Gain2 : Gain  Gain=BLn  Multiplication=Matrix(K*u)
  Gain3 : Gain  Gain=DLn  Multiplication=Matrix(K*u)
  Gain4 : Gain  Gain=CLn  Multiplication=Matrix(K*u)
  Gain5 : Gain  Gain=L  Multiplication=Matrix(K*u)
  Integrator : Integrator
  Subtract1 : Sum  Inputs=+++
  Subtract2 : Sum
  Subtract3 : Sum  Inputs=+-
  Est : Outport
  wires:
  Integrator/1 -> Est/1, Gain1/1, Gain4/1
  Gain2/1 -> Subtract1/1
  Gain4/1 -> Subtract2/2
  Gain3/1 -> Subtract2/1
  U/1 -> Gain3/1, Gain2/1
  Y/1 -> Subtract3/1
  Subtract2/1 -> Subtract3/2
  Subtract3/1 -> Gain5/1
  Gain1/1 -> Subtract1/3
  Gain5/1 -> Subtract1/2
  Subtract1/1 -> Integrator/1

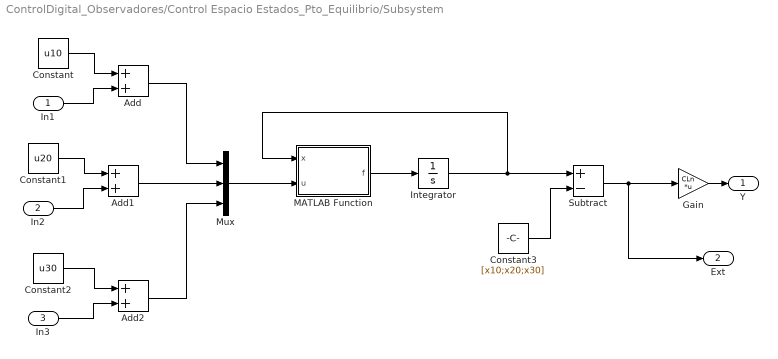
== system ControlDigital_Observadores/Control Espacio Estados_Pto_Equilibrio/Subsystem ==
  In1 : Inport
  In2 : Inport  Port=2
  In3 : Inport  Port=3
  Add : Sum
  Add1 : Sum
  Add2 : Sum
  Constant : Constant  Value=u10
  Constant1 : Constant  Value=u20
  Constant2 : Constant  Value=u30
  Constant3 : Constant  Value=[x10;x20;x30]
  Gain : Gain  Gain=CLn  Multiplication=Matrix(K*u)
  Integrator : Integrator  InitialCondition=[x10;x20;x30]+xini
  MATLAB Function : MATLAB Function  TreatAsAtomicUnit=on
  Mux : Mux  Inputs=3
  Subtract : Sum  Inputs=+-
  Y : Outport
  Ext : Outport  Port=2
  wires:
  Subtract/1 -> Ext/1, Gain/1
  Gain/1 -> Y/1
  In1/1 -> Add/2
  Constant/1 -> Add/1
  Add/1 -> Mux/1
  Constant1/1 -> Add1/1
  Add1/1 -> Mux/2
  Mux/1 -> MATLAB Function/2(u)
  Integrator/1 -> MATLAB Function/1(x), Subtract/1
  MATLAB Function/1(f) -> Integrator/1
  In2/1 -> Add1/2
  In3/1 -> Add2/2
  Constant2/1 -> Add2/1
  Constant3/1 -> Subtract/2
  Add2/1 -> Mux/3

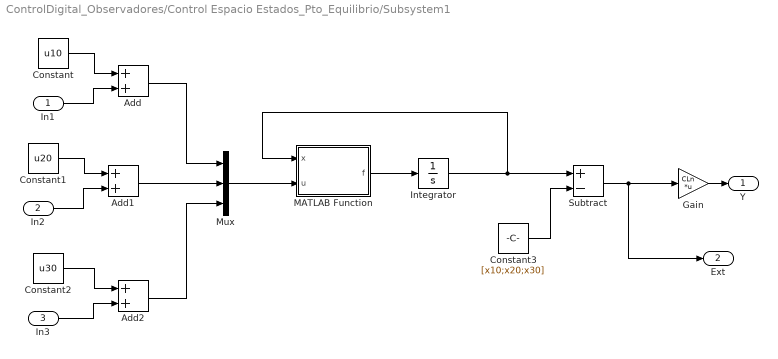
== system ControlDigital_Observadores/Control Espacio Estados_Pto_Equilibrio/Subsystem1 ==
  In1 : Inport
  In2 : Inport  Port=2
  In3 : Inport  Port=3
  Add : Sum
  Add1 : Sum
  Add2 : Sum
  Constant : Constant  Value=u10
  Constant1 : Constant  Value=u20
  Constant2 : Constant  Value=u30
  Constant3 : Constant  Value=[x10;x20;x30]
  Gain : Gain  Gain=CLn  Multiplication=Matrix(K*u)
  Integrator : Integrator  InitialCondition=[x10;x20;x30]+xini
  MATLAB Function : MATLAB Function  TreatAsAtomicUnit=on
  Mux : Mux  Inputs=3
  Subtract : Sum  Inputs=+-
  Y : Outport
  Ext : Outport  Port=2
  wires:
  Subtract/1 -> Ext/1, Gain/1
  Gain/1 -> Y/1
  In1/1 -> Add/2
  Constant/1 -> Add/1
  Add/1 -> Mux/1
  Constant1/1 -> Add1/1
  Add1/1 -> Mux/2
  Mux/1 -> MATLAB Function/2(u)
  Integrator/1 -> MATLAB Function/1(x), Subtract/1
  MATLAB Function/1(f) -> Integrator/1
  In2/1 -> Add1/2
  In3/1 -> Add2/2
  Constant2/1 -> Add2/1
  Constant3/1 -> Subtract/2
  Add2/1 -> Mux/3

== system ControlDigital_Observadores/Control Espacio Estados_Pto_Equilibrio/Subsystem2 ==
  U : Inport
  Y : Inport  Port=2
  Gain1 : Gain  Gain=ALn  Multiplication=Matrix(K*u)
  Gain2 : Gain  Gain=BLn  Multiplication=Matrix(K*u)
  Gain3 : Gain  Gain=DLn  Multiplication=Matrix(K*u)
  Gain4 : Gain  Gain=CLn  Multiplication=Matrix(K*u)
  Gain5 : Gain  Gain=L  Multiplication=Matrix(K*u)
  Integrator : Integrator
  Subtract1 : Sum  Inputs=+++
  Subtract2 : Sum
  Subtract3 : Sum  Inputs=+-
  Est : Outport
  wires:
  Integrator/1 -> Est/1, Gain1/1, Gain4/1
  Gain2/1 -> Subtract1/1
  Gain4/1 -> Subtract2/2
  Gain3/1 -> Subtract2/1
  U/1 -> Gain3/1, Gain2/1
  Y/1 -> Subtract3/1
  Subtract2/1 -> Subtract3/2
  Subtract3/1 -> Gain5/1
  Gain1/1 -> Subtract1/3
  Gain5/1 -> Subtract1/2
  Subtract1/1 -> Integrator/1

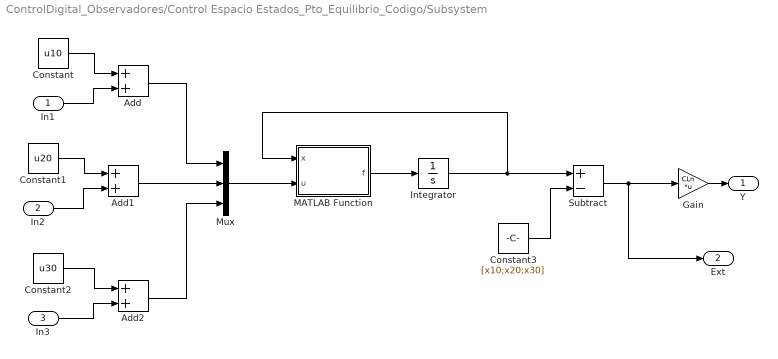
== system ControlDigital_Observadores/Control Espacio Estados_Pto_Equilibrio_Codigo/Subsystem ==
  In1 : Inport
  In2 : Inport  Port=2
  In3 : Inport  Port=3
  Add : Sum
  Add1 : Sum
  Add2 : Sum
  Constant : Constant  Value=u10
  Constant1 : Constant  Value=u20
  Constant2 : Constant  Value=u30
  Constant3 : Constant  Value=[x10;x20;x30]
  Gain : Gain  Gain=CLn  Multiplication=Matrix(K*u)
  Integrator : Integrator  InitialCondition=[x10;x20;x30]+xini
  MATLAB Function : MATLAB Function  TreatAsAtomicUnit=on
  Mux : Mux  Inputs=3
  Subtract : Sum  Inputs=+-
  Y : Outport
  Ext : Outport  Port=2
  wires:
  Subtract/1 -> Ext/1, Gain/1
  Gain/1 -> Y/1
  In1/1 -> Add/2
  Constant/1 -> Add/1
  Add/1 -> Mux/1
  Constant1/1 -> Add1/1
  Add1/1 -> Mux/2
  Mux/1 -> MATLAB Function/2(u)
  Integrator/1 -> MATLAB Function/1(x), Subtract/1
  MATLAB Function/1(f) -> Integrator/1
  In2/1 -> Add1/2
  In3/1 -> Add2/2
  Constant2/1 -> Add2/1
  Constant3/1 -> Subtract/2
  Add2/1 -> Mux/3

== system ControlDigital_Observadores/Control Espacio Estados_Pto_Equilibrio_Codigo/Subsystem1 ==
  In1 : Inport
  In2 : Inport  Port=2
  In3 : Inport  Port=3
  Add : Sum
  Add1 : Sum
  Add2 : Sum
  Constant : Constant  Value=u10
  Constant1 : Constant  Value=u20
  Constant2 : Constant  Value=u30
  Constant3 : Constant  Value=[x10;x20;x30]
  Gain : Gain  Gain=CLn  Multiplication=Matrix(K*u)
  Integrator : Integrator  InitialCondition=[x10;x20;x30]+xini
  MATLAB Function : MATLAB Function  TreatAsAtomicUnit=on
  Mux : Mux  Inputs=3
  Subtract : Sum  Inputs=+-
  Y : Outport
  Ext : Outport  Port=2
  wires:
  Subtract/1 -> Ext/1, Gain/1
  Gain/1 -> Y/1
  In1/1 -> Add/2
  Constant/1 -> Add/1
  Add/1 -> Mux/1
  Constant1/1 -> Add1/1
  Add1/1 -> Mux/2
  Mux/1 -> MATLAB Function/2(u)
  Integrator/1 -> MATLAB Function/1(x), Subtract/1
  MATLAB Function/1(f) -> Integrator/1
  In2/1 -> Add1/2
  In3/1 -> Add2/2
  Constant2/1 -> Add2/1
  Constant3/1 -> Subtract/2
  Add2/1 -> Mux/3

== system ControlDigital_Observadores/Control Espacio Estados_Pto_Equilibrio_Codigo/Subsystem2 ==
  U : Inport
  Y : Inport  Port=2
  Gain1 : Gain  Gain=ALn  Multiplication=Matrix(K*u)
  Gain2 : Gain  Gain=BLn  Multiplication=Matrix(K*u)
  Gain3 : Gain  Gain=DLn  Multiplication=Matrix(K*u)
  Gain4 : Gain  Gain=CLn  Multiplication=Matrix(K*u)
  Gain5 : Gain  Gain=L  Multiplication=Matrix(K*u)
  Integrator : Integrator
  Subtract1 : Sum  Inputs=+++
  Subtract2 : Sum
  Subtract3 : Sum  Inputs=+-
  Est : Outport
  wires:
  Integrator/1 -> Est/1, Gain1/1, Gain4/1
  Gain2/1 -> Subtract1/1
  Gain4/1 -> Subtract2/2
  Gain3/1 -> Subtract2/1
  U/1 -> Gain3/1, Gain2/1
  Y/1 -> Subtract3/1
  Subtract2/1 -> Subtract3/2
  Subtract3/1 -> Gain5/1
  Gain1/1 -> Subtract1/3
  Gain5/1 -> Subtract1/2
  Subtract1/1 -> Integrator/1

== system ControlDigital_Observadores/Control Espacio Unificado_Continua/Subsystem ==
  In1 : Inport
  In2 : Inport  Port=2
  In3 : Inport  Port=3
  Add : Sum
  Add1 : Sum
  Add2 : Sum
  Constant : Constant  Value=u10
  Constant1 : Constant  Value=u20
  Constant2 : Constant  Value=u30
  Constant3 : Constant  Value=[x10;x20;x30]
  Gain : Gain  Gain=CLn  Multiplication=Matrix(K*u)
  Integrator : Integrator  InitialCondition=[x10;x20;x30]
  MATLAB Function : MATLAB Function  TreatAsAtomicUnit=on
  Mux : Mux  Inputs=3
  Subtract : Sum  Inputs=+-
  Y : Outport
  Ext : Outport  Port=2
  wires:
  Subtract/1 -> Ext/1, Gain/1
  Gain/1 -> Y/1
  In1/1 -> Add/2
  Constant/1 -> Add/1
  Add/1 -> Mux/1
  Constant1/1 -> Add1/1
  Add1/1 -> Mux/2
  Mux/1 -> MATLAB Function/2(u)
  Integrator/1 -> MATLAB Function/1(x), Subtract/1
  MATLAB Function/1(f) -> Integrator/1
  In2/1 -> Add1/2
  In3/1 -> Add2/2
  Constant2/1 -> Add2/1
  Constant3/1 -> Subtract/2
  Add2/1 -> Mux/3

== system ControlDigital_Observadores/Control Espacio Unificado_Continua/Subsystem1 ==
  In1 : Inport
  Gain1 : Gain  Gain=ALn  Multiplication=Matrix(K*u)
  Gain2 : Gain  Gain=BLn  Multiplication=Matrix(K*u)
  Gain3 : Gain  Gain=DLn  Multiplication=Matrix(K*u)
  Gain4 : Gain  Gain=CLn  Multiplication=Matrix(K*u)
  Integrator : Integrator
  Subtract1 : Sum
  Subtract2 : Sum
  Y_L : Outport
  Ext_L : Outport  Port=2
  wires:
  Subtract2/1 -> Y_L/1
  Subtract1/1 -> Integrator/1
  Integrator/1 -> Ext_L/1, Gain1/1, Gain4/1
  Gain1/1 -> Subtract1/2
  Gain2/1 -> Subtract1/1
  Gain4/1 -> Subtract2/2
  Gain3/1 -> Subtract2/1
  In1/1 -> Gain3/1, Gain2/1

== system ControlDigital_Observadores/Control Espacio Unificado_Discreto/Subsystem ==
  In1 : Inport
  In2 : Inport  Port=2
  In3 : Inport  Port=3
  Add : Sum
  Add1 : Sum
  Add2 : Sum
  Constant : Constant  Value=u10
  Constant1 : Constant  Value=u20
  Constant2 : Constant  Value=u30
  Constant3 : Constant  Value=[x10;x20;x30]
  Gain : Gain  Gain=CLn  Multiplication=Matrix(K*u)
  Integrator : Integrator  InitialCondition=[x10;x20;x30]
  MATLAB Function : MATLAB Function  TreatAsAtomicUnit=on
  Mux : Mux  Inputs=3
  Subtract : Sum  Inputs=+-
  Y : Outport
  Ext : Outport  Port=2
  wires:
  Subtract/1 -> Ext/1, Gain/1
  Gain/1 -> Y/1
  In1/1 -> Add/2
  Constant/1 -> Add/1
  Add/1 -> Mux/1
  Constant1/1 -> Add1/1
  Add1/1 -> Mux/2
  Mux/1 -> MATLAB Function/2(u)
  Integrator/1 -> MATLAB Function/1(x), Subtract/1
  MATLAB Function/1(f) -> Integrator/1
  In2/1 -> Add1/2
  In3/1 -> Add2/2
  Constant2/1 -> Add2/1
  Constant3/1 -> Subtract/2
  Add2/1 -> Mux/3

== system ControlDigital_Observadores/Control Espacio Unificado_Discreto/Subsystem1 ==
  In1 : Inport
  Gain1 : Gain  Gain=ALn  Multiplication=Matrix(K*u)
  Gain2 : Gain  Gain=BLn  Multiplication=Matrix(K*u)
  Gain3 : Gain  Gain=DLn  Multiplication=Matrix(K*u)
  Gain4 : Gain  Gain=CLn  Multiplication=Matrix(K*u)
  Integrator : Integrator
  Subtract1 : Sum
  Subtract2 : Sum
  Y_L : Outport
  Ext_L : Outport  Port=2
  wires:
  Subtract2/1 -> Y_L/1
  Subtract1/1 -> Integrator/1
  Integrator/1 -> Ext_L/1, Gain1/1, Gain4/1
  Gain1/1 -> Subtract1/2
  Gain2/1 -> Subtract1/1
  Gain4/1 -> Subtract2/2
  Gain3/1 -> Subtract2/1
  In1/1 -> Gain3/1, Gain2/1

== system ControlDigital_Observadores/Control Espacio Unificado_Discreto_codigo/Subsystem ==
  In1 : Inport
  In2 : Inport  Port=2
  In3 : Inport  Port=3
  Add : Sum
  Add1 : Sum
  Add2 : Sum
  Constant : Constant  Value=u10
  Constant1 : Constant  Value=u20
  Constant2 : Constant  Value=u30
  Constant3 : Constant  Value=[x10;x20;x30]
  Gain : Gain  Gain=CLn  Multiplication=Matrix(K*u)
  Integrator : Integrator  InitialCondition=[x10;x20;x30]
  MATLAB Function : MATLAB Function  TreatAsAtomicUnit=on
  Mux : Mux  Inputs=3
  Subtract : Sum  Inputs=+-
  Y : Outport
  Ext : Outport  Port=2
  wires:
  Subtract/1 -> Ext/1, Gain/1
  Gain/1 -> Y/1
  In1/1 -> Add/2
  Constant/1 -> Add/1
  Add/1 -> Mux/1
  Constant1/1 -> Add1/1
  Add1/1 -> Mux/2
  Mux/1 -> MATLAB Function/2(u)
  Integrator/1 -> MATLAB Function/1(x), Subtract/1
  MATLAB Function/1(f) -> Integrator/1
  In2/1 -> Add1/2
  In3/1 -> Add2/2
  Constant2/1 -> Add2/1
  Constant3/1 -> Subtract/2
  Add2/1 -> Mux/3

== system ControlDigital_Observadores/Control Espacio Unificado_Discreto_codigo/Subsystem1 ==
  In1 : Inport
  Gain1 : Gain  Gain=ALn  Multiplication=Matrix(K*u)
  Gain2 : Gain  Gain=BLn  Multiplication=Matrix(K*u)
  Gain3 : Gain  Gain=DLn  Multiplication=Matrix(K*u)
  Gain4 : Gain  Gain=CLn  Multiplication=Matrix(K*u)
  Integrator : Integrator
  Subtract1 : Sum
  Subtract2 : Sum
  Y_L : Outport
  Ext_L : Outport  Port=2
  wires:
  Subtract2/1 -> Y_L/1
  Subtract1/1 -> Integrator/1
  Integrator/1 -> Ext_L/1, Gain1/1, Gain4/1
  Gain1/1 -> Subtract1/2
  Gain2/1 -> Subtract1/1
  Gain4/1 -> Subtract2/2
  Gain3/1 -> Subtract2/1
  In1/1 -> Gain3/1, Gain2/1

== system ControlDigital_Observadores/Control Espacio Unificado_Funcion LQG/Subsystem ==
  In1 : Inport
  In2 : Inport  Port=2
  In3 : Inport  Port=3
  Add : Sum
  Add1 : Sum
  Add2 : Sum
  Constant : Constant  Value=u10
  Constant1 : Constant  Value=u20
  Constant2 : Constant  Value=u30
  Constant3 : Constant  Value=[x10;x20;x30]
  Gain : Gain  Gain=CLn  Multiplication=Matrix(K*u)
  Integrator : Integrator  InitialCondition=[x10;x20;x30]
  MATLAB Function : MATLAB Function  TreatAsAtomicUnit=on
  Mux : Mux  Inputs=3
  Subtract : Sum  Inputs=+-
  Y : Outport
  Ext : Outport  Port=2
  wires:
  Subtract/1 -> Ext/1, Gain/1
  Gain/1 -> Y/1
  In1/1 -> Add/2
  Constant/1 -> Add/1
  Add/1 -> Mux/1
  Constant1/1 -> Add1/1
  Add1/1 -> Mux/2
  Mux/1 -> MATLAB Function/2(u)
  Integrator/1 -> MATLAB Function/1(x), Subtract/1
  MATLAB Function/1(f) -> Integrator/1
  In2/1 -> Add1/2
  In3/1 -> Add2/2
  Constant2/1 -> Add2/1
  Constant3/1 -> Subtract/2
  Add2/1 -> Mux/3

== system ControlDigital_Observadores/Control Espacio Unificado_Funcion LQG/Subsystem1 ==
  In1 : Inport
  In2 : Inport  Port=2
  In3 : Inport  Port=3
  Add : Sum
  Add1 : Sum
  Add2 : Sum
  Constant : Constant  Value=u10
  Constant1 : Constant  Value=u20
  Constant2 : Constant  Value=u30
  Constant3 : Constant  Value=[x10;x20;x30]
  Gain : Gain  Gain=CLn  Multiplication=Matrix(K*u)
  Integrator : Integrator  InitialCondition=[x10;x20;x30]
  MATLAB Function : MATLAB Function  TreatAsAtomicUnit=on
  Mux : Mux  Inputs=3
  Subtract : Sum  Inputs=+-
  Y : Outport
  Ext : Outport  Port=2
  wires:
  Subtract/1 -> Ext/1, Gain/1
  Gain/1 -> Y/1
  In1/1 -> Add/2
  Constant/1 -> Add/1
  Add/1 -> Mux/1
  Constant1/1 -> Add1/1
  Add1/1 -> Mux/2
  Mux/1 -> MATLAB Function/2(u)
  Integrator/1 -> MATLAB Function/1(x), Subtract/1
  MATLAB Function/1(f) -> Integrator/1
  In2/1 -> Add1/2
  In3/1 -> Add2/2
  Constant2/1 -> Add2/1
  Constant3/1 -> Subtract/2
  Add2/1 -> Mux/3

== matlab function ControlDigital_Observadores/Control Espacio Unificado_Continua/Subsystem/MATLAB Function ==
  data: x input; u input; f output
function f = fcn(x,u)

a = 2;
b = 4;
c = 1;
d = 3;

x1 = x(1);
x2 = x(2);
x3 = x(3);
u1 = u(1);
u2 = u(2);
u3 = u(3);

f1 = -a*x2 - b*x1^2 + u1*u2;
f2 = -c*x3*x2 + u2^2 ;
f3 = -d*x3 + u3*x1 + u1;

f = [f1;f2;f3];

== matlab function ControlDigital_Observadores/Control Espacio Estados_Observador/Subsystem/MATLAB Function ==
  data: x input; u input; f output
function f = fcn(x,u)

a = 2;
b = 4;
c = 1;
d = 3;

x1 = x(1);
x2 = x(2);
x3 = x(3);
u1 = u(1);
u2 = u(2);
u3 = u(3);

f1 = -a*x2 - b*x1^2 + u1*u2;
f2 = -c*x3*x2 + u2^2 ;
f3 = -d*x3 + u3*x1 + u1;

f = [f1;f2;f3];

== matlab function ControlDigital_Observadores/Control Espacio Unificado_Discreto/Subsystem/MATLAB Function ==
  data: x input; u input; f output
function f = fcn(x,u)

a = 2;
b = 4;
c = 1;
d = 3;

x1 = x(1);
x2 = x(2);
x3 = x(3);
u1 = u(1);
u2 = u(2);
u3 = u(3);

f1 = -a*x2 - b*x1^2 + u1*u2;
f2 = -c*x3*x2 + u2^2 ;
f3 = -d*x3 + u3*x1 + u1;

f = [f1;f2;f3];

== matlab function ControlDigital_Observadores/Control Espacio Unificado_Funcion LQG/Subsystem/MATLAB Function ==
  data: x input; u input; f output
function f = fcn(x,u)

a = 2;
b = 4;
c = 1;
d = 3;

x1 = x(1);
x2 = x(2);
x3 = x(3);
u1 = u(1);
u2 = u(2);
u3 = u(3);

f1 = -a*x2 - b*x1^2 + u1*u2;
f2 = -c*x3*x2 + u2^2 ;
f3 = -d*x3 + u3*x1 + u1;

f = [f1;f2;f3];

== matlab function ControlDigital_Observadores/Control Espacio Unificado_Funcion LQG/Subsystem1/MATLAB Function ==
  data: x input; u input; f output
function f = fcn(x,u)

a = 2;
b = 4;
c = 1;
d = 3;

x1 = x(1);
x2 = x(2);
x3 = x(3);
u1 = u(1);
u2 = u(2);
u3 = u(3);

f1 = -a*x2 - b*x1^2 + u1*u2;
f2 = -c*x3*x2 + u2^2 ;
f3 = -d*x3 + u3*x1 + u1;

f = [f1;f2;f3];

== matlab function ControlDigital_Observadores/Control Espacio Estados_Pto_Equilibrio/Subsystem/MATLAB Function ==
  data: x input; u input; f output
function f = fcn(x,u)

a = 2;
b = 4;
c = 1;
d = 3;

x1 = x(1);
x2 = x(2);
x3 = x(3);
u1 = u(1);
u2 = u(2);
u3 = u(3);

f1 = -a*x2 - b*x1^2 + u1*u2;
f2 = -c*x3*x2 + u2^2 ;
f3 = -d*x3 + u3*x1 + u1;

f = [f1;f2;f3];

== matlab function ControlDigital_Observadores/Control Espacio Estados_Pto_Equilibrio/Subsystem1/MATLAB Function ==
  data: x input; u input; f output
function f = fcn(x,u)

a = 2;
b = 4;
c = 1;
d = 3;

x1 = x(1);
x2 = x(2);
x3 = x(3);
u1 = u(1);
u2 = u(2);
u3 = u(3);

f1 = -a*x2 - b*x1^2 + u1*u2;
f2 = -c*x3*x2 + u2^2 ;
f3 = -d*x3 + u3*x1 + u1;

f = [f1;f2;f3];

== matlab function ControlDigital_Observadores/Control Espacio Unificado_Discreto_codigo/Subsystem/MATLAB Function ==
  data: x input; u input; f output
function f = fcn(x,u)

a = 2;
b = 4;
c = 1;
d = 3;

x1 = x(1);
x2 = x(2);
x3 = x(3);
u1 = u(1);
u2 = u(2);
u3 = u(3);

f1 = -a*x2 - b*x1^2 + u1*u2;
f2 = -c*x3*x2 + u2^2 ;
f3 = -d*x3 + u3*x1 + u1;

f = [f1;f2;f3];

== matlab function ControlDigital_Observadores/Control Espacio Estados_Pto_Equilibrio_Codigo/Subsystem/MATLAB Function ==
  data: x input; u input; f output
function f = fcn(x,u)

a = 2;
b = 4;
c = 1;
d = 3;

x1 = x(1);
x2 = x(2);
x3 = x(3);
u1 = u(1);
u2 = u(2);
u3 = u(3);

f1 = -a*x2 - b*x1^2 + u1*u2;
f2 = -c*x3*x2 + u2^2 ;
f3 = -d*x3 + u3*x1 + u1;

f = [f1;f2;f3];

== matlab function ControlDigital_Observadores/Control Espacio Unificado_Discreto_codigo/MATLAB Function1 ==
  data: Sp input; U output; Pv input; Con_ini input; Con_out output
function [U,Con_out] = fcn(Sp,Pv,Con_ini)

xk_1 = Con_ini;
Gc = [0.746610612948490 -0.103501443891891 -0.0404324705771849 0.812299293177354 0.141849092232024;-0.0603433539177371 0.790323271392663 -0.0252718557409297 0.393897732028220 0.0479395314225843;0.00718824100196412 0.00697734161963191 0.900848611102580 0.0446591934243858 0.210425736705796;0 0 0 1 0;0 0 0 0 1];
Hsp = [0.00430844185632985 0.000758682012549799;0.00210250662629489 0.000264124852434563;0.000218128628657280 0.00106895139663100;0.0100000000000000 0;0 0.0100000000000000];
Hpv = [0.000479486167369631 -0.000288972451095416;-0.00238157201735919 -0.000881111070239073;0.00294110392637133 3.25906964414870e-05;-0.0100000000000000 0;0 -0.0100000000000000];
Cc = [-1.81824484654282 0.883331520825385 -1.41121305570245 15.2661814521523 3.14296545851546;-0.984003410318051 -2.50472404587341 0.0931967286183644 5.98781852266087 0.795818253049450;0.0294205084155260 0.00123380084294658 -2.94010814506701 -5.57581681995041 9.45983305532884];
U = Cc*xk_1;
xk = Gc*xk_1 + Hsp*Sp + Hpv*Pv;
xk_1 = xk;
Con_out = [xk_1];

== matlab function ControlDigital_Observadores/Control Espacio Estados_Pto_Equilibrio_Codigo/Subsystem1/MATLAB Function ==
  data: x input; u input; f output
function f = fcn(x,u)

a = 2;
b = 4;
c = 1;
d = 3;

x1 = x(1);
x2 = x(2);
x3 = x(3);
u1 = u(1);
u2 = u(2);
u3 = u(3);

f1 = -a*x2 - b*x1^2 + u1*u2;
f2 = -c*x3*x2 + u2^2 ;
f3 = -d*x3 + u3*x1 + u1;

f = [f1;f2;f3];

== matlab function ControlDigital_Observadores/Control Espacio Estados_Pto_Equilibrio_Codigo/MATLAB Function1 ==
  data: U output; Pv input; Con_ini input; Con_out output
function [U,Con_out] = fcn(Pv,Con_ini)

xk_1 = Con_ini;
Gc = [0.219622954373264 -0.0162427489226351 -0.124142100484963;-0.00216885601277124 0.941730193377791 -0.00884447579451413;-0.103514912910946 0.00365266521117835 0.571576442259887];
Hc = [0.691929116431979 0.113125989978681;-0.00293756889568736 -0.0380241558989840;0.136252869442036 0.390469801888981];
Cc = [-0.136059231929892 0.0548143529839082 -0.637527605041404;-0.0675442603585678 -0.251022668037956 -0.107663526273814;-0.112997617923268 0.0578323318739971 -0.823064738389738];
U = Cc*xk_1;
xk = Gc*xk_1 + Hc*Pv;
xk_1 = xk;
Con_out = [xk_1];
